simulink model "LQRCalcs_model"  (R2022a)
settings: Solver=VariableStepAuto  StartTime=0.0  StopTime=10.0  RelTol=1e-3
values from neighbouring files (symbols this model uses):
  Aa = [0 1 0 0 0 0 ... (first row only)    [LQRCalcs.m]
  Ap = [0 1 0 0 0 0 ... (first row only)    [LQRCalcs.m]
  b = 1    [LQRCalcs.m]
  Ba = [0 0 0 0 ... (first row only)    [LQRCalcs.m]
  Bp = [0 0 0 ... (first row only)    [LQRCalcs.m]
  g = -9.81    [LQRCalcs.m]    (also in cf_firstOrderStateMdl.m = 9.81; init_parameters.m = 9.81; main.m = 9.81; parameters_buildingSimulink.m = 9.81)
  m = 0.5    [LQRCalcs.m]    (also in cf_firstOrderStateMdl.m = 0.003; init_parameters.m = 4.34; main.m = 4.34; parameters_buildingSimulink.m = 4.34)
undefined symbols (not defined in the file or in its folder): Kp
libraries: sharedtransform x1, uavutilslib x1
settings Model: Creator=Drew Lab Computer 1  LastModifiedBy=Drew Lab Computer 1

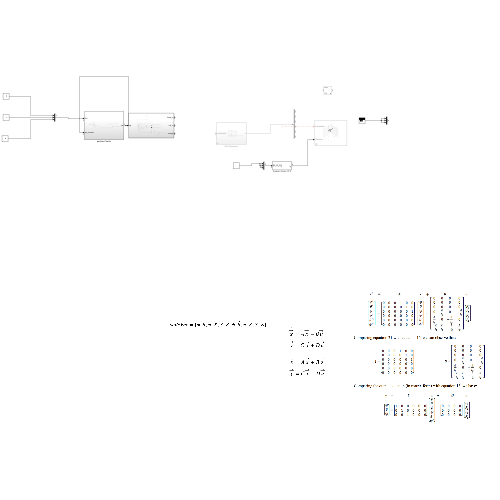
[thumbnail: Simulink's stored preview of the top-level diagram]
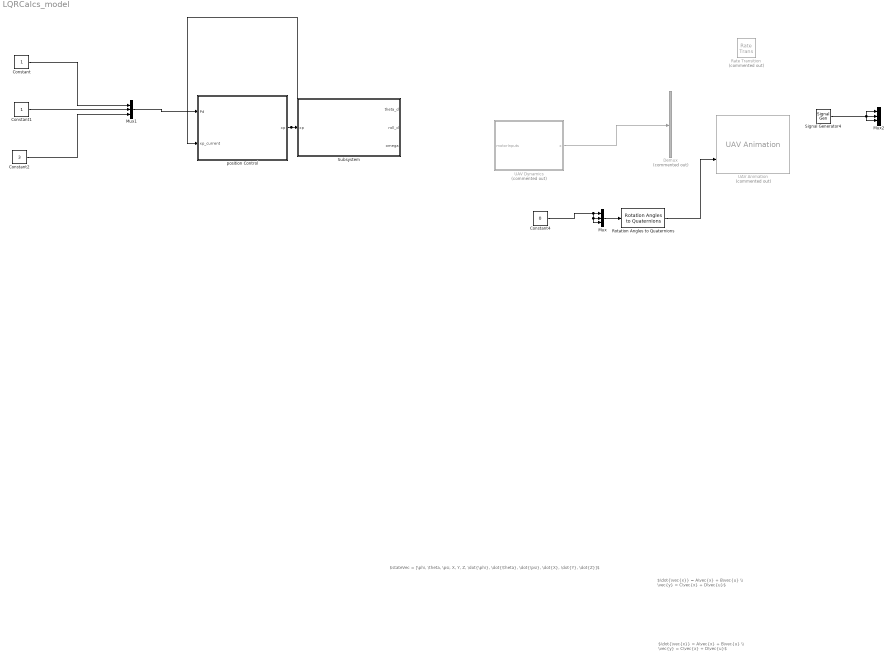
== system LQRCalcs_model ==
  note: $\dot{\vec{x}} = A\vec{x} + B\vec{u} \\ \vec{y} = C\vec{x} + D\vec{u}$
  note: $stateVec = [\phi, \theta, \psi, X, Y, Z, \dot{\phi}, \dot{\theta}, \dot{\psi}, \dot{X}, \dot{Y}, \dot{Z}]$
  note: $\dot{\vec{x}} = A\vec{x} + B\vec{u} \\ \vec{y} = C\vec{x} + D\vec{u}$
  Constant : Constant
  Constant1 : Constant
  Constant2 : Constant  Value=3
  Constant4 : Constant  Value=0
  Demux : Demux  Commented=on  Outputs=6
  Mux : Mux  Inputs=3
  Mux1 : Mux  Inputs=3
  Mux2 : Mux  Inputs=3
  Rate Transition : RateTransition  Commented=on  OutPortSampleTime=t_sampling
  Rotation Angles to Quaternions : sharedtransform/Rotation Angles to Quaternions  rotationOrder=ZYX  aMode=aMode
      settings: SourceProductBaseCode=AE,PW,DR,MT,VE
  Signal Generator4 : SignalGenerator  Amplitude=0  Units=rad/sec
  Subsystem : Subsystem
  UAV Animation : uavutilslib/UAV Animation  Commented=on  UAVType=Multirotor  UAVSize=1  InertialZDirection=Down  SampleTime=-1
      settings: SourceProductBaseCode=UV
  UAV Dynamics : Subsystem  Commented=on
  position Control : Subsystem
  wires:
  Signal Generator4/1 -> Mux2/1, Mux2/3, Mux2/2
  UAV Dynamics/1(x) -> Demux/1
  position Control/1(xp) -> position Control/2(xp_current), Subsystem/1(xp)
  Mux/1 -> Rotation Angles to Quaternions/1
  Constant4/1 -> Mux/3, Mux/2, Mux/1
  Rotation Angles to Quaternions/1 -> UAV Animation/2
  ? -> UAV Animation/1
  Constant1/1 -> Mux1/2
  Constant/1 -> Mux1/1
  Constant2/1 -> Mux1/3
  Mux1/1 -> position Control/1(Pd)

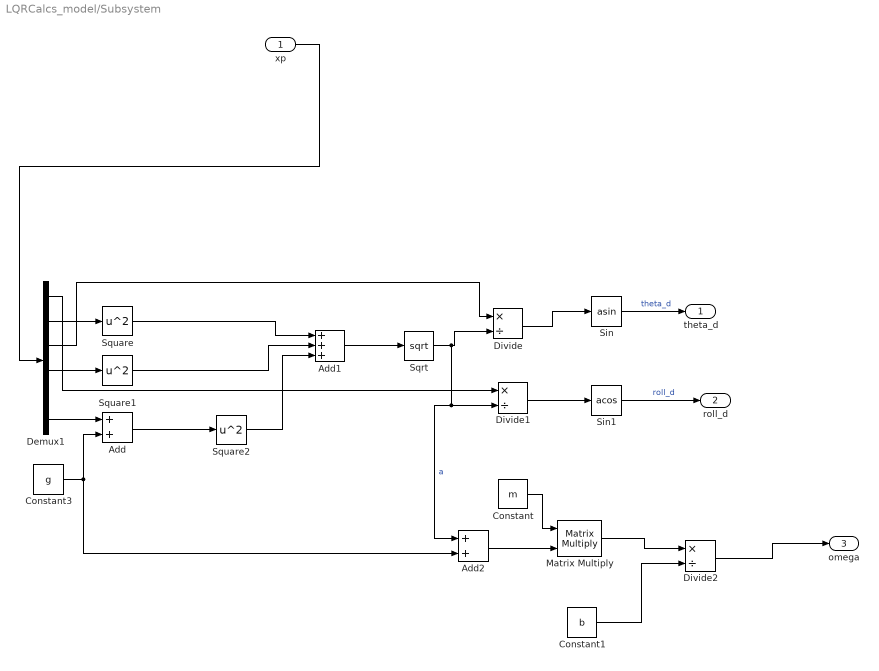
== system LQRCalcs_model/Subsystem ==
  xp : Inport
  Add : Sum
  Add1 : Sum  Inputs=+++
  Add2 : Sum
  Constant : Constant  Value=m
  Constant1 : Constant  Value=b
  Constant3 : Constant  Value=g
  Demux1 : Demux  Outputs=6
  Divide : Product  Inputs=*/
  Divide1 : Product  Inputs=*/
  Divide2 : Product  Inputs=*/
  Matrix Multiply : Product  Multiplication=Matrix(*)
  Sin : Trigonometry  Operator=asin
  Sin1 : Trigonometry  Operator=acos
  Sqrt : Sqrt
  Square : Math  Operator=square
  Square1 : Math  Operator=square
  Square2 : Math  Operator=square
  theta_d : Outport
  roll_d : Outport  Port=2
  omega : Outport  Port=3
  wires:
  Square2/1 -> Add1/3
  Constant3/1 -> Add/2, Add2/2
  Divide/1 -> Sin/1
  Square1/1 -> Add1/2
  Demux1/1 -> Divide1/1
  Square/1 -> Add1/1
  Demux1/6 -> Add/1
  Sqrt/1 -> Divide1/2, Add2/1, Divide/2  "a"
  Add1/1 -> Sqrt/1
  Add/1 -> Square2/1
  Demux1/4 -> Square1/1
  Demux1/2 -> Square/1
  Divide1/1 -> Sin1/1
  Demux1/3 -> Divide/1
  Sin/1 -> theta_d/1  "theta_d"
  xp/1 -> Demux1/1
  Sin1/1 -> roll_d/1  "roll_d"
  Constant/1 -> Matrix Multiply/1
  Add2/1 -> Matrix Multiply/2
  Matrix Multiply/1 -> Divide2/1
  Constant1/1 -> Divide2/2
  Divide2/1 -> omega/1

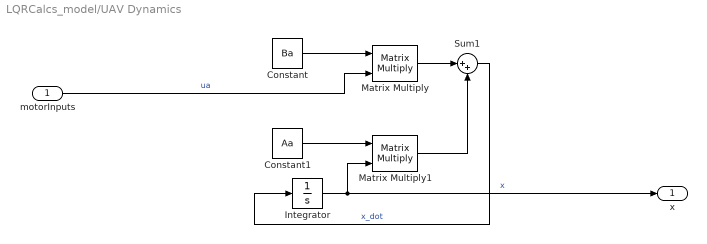
== system LQRCalcs_model/UAV Dynamics ==
  motorInputs : Inport
  Constant : Constant  Value=Ba
  Constant1 : Constant  Value=Aa
  Integrator : Integrator
  Matrix Multiply : Product  Multiplication=Matrix(*)
  Matrix Multiply1 : Product  Multiplication=Matrix(*)
  Sum1 : Sum  Inputs=|++
  x : Outport
  wires:
  Sum1/1 -> Integrator/1  "x_dot"
  Matrix Multiply1/1 -> Sum1/2
  Constant/1 -> Matrix Multiply/1
  motorInputs/1 -> Matrix Multiply/2  "ua"
  Integrator/1 -> Matrix Multiply1/2, x/1  "x"
  Matrix Multiply/1 -> Sum1/1
  Constant1/1 -> Matrix Multiply1/1

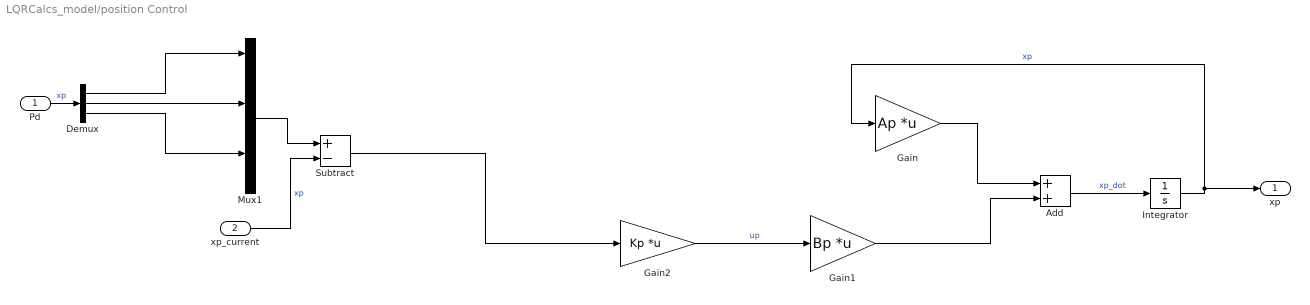
== system LQRCalcs_model/position Control ==
  Pd : Inport
  xp_current : Inport  Port=2
  Add : Sum
  Demux : Demux  Outputs=3
  Gain : Gain  Gain=Ap  Multiplication=Matrix(K*u)
  Gain1 : Gain  Gain=Bp  Multiplication=Matrix(K*u)
  Gain2 : Gain  Gain=Kp  Multiplication=Matrix(K*u)
  Integrator : Integrator
  Mux1 : Mux  Inputs=6
  Subtract : Sum  Inputs=+-
  xp : Outport
  wires:
  Add/1 -> Integrator/1  "xp_dot"
  Gain1/1 -> Add/2
  Gain/1 -> Add/1
  Integrator/1 -> xp/1, Gain/1  "xp"
  Gain2/1 -> Gain1/1  "up"
  xp_current/1 -> Subtract/2  "xp"
  Subtract/1 -> Gain2/1
  Pd/1 -> Demux/1  "xp"
  Demux/1 -> Mux1/1
  Demux/2 -> Mux1/3
  Demux/3 -> Mux1/5
  Mux1/1 -> Subtract/1
